simulink model "rev1_PEM"  (R2024a)
settings: Solver=VariableStepAuto  StartTime=0.0  StopTime=10.0  RelTol=1e-3
libraries: spsDiodeLib x2, spsGroundLib x2, spsParallelRLCBranchLib x1, spsControlledVoltageSourceLib x1, spsVariableResistorLib x1
settings Model: Creator=ADMIN  LastModifiedBy=ADMIN

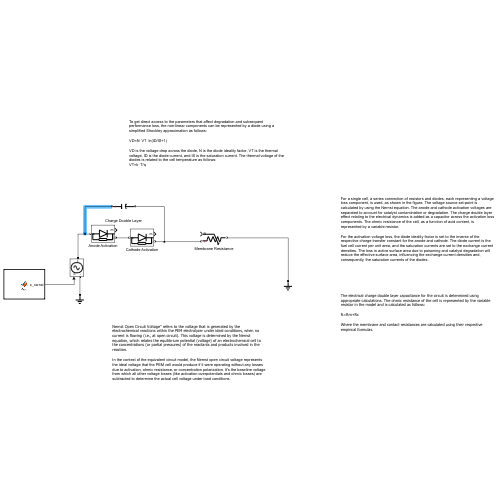
[thumbnail: Simulink's stored preview of the top-level diagram]
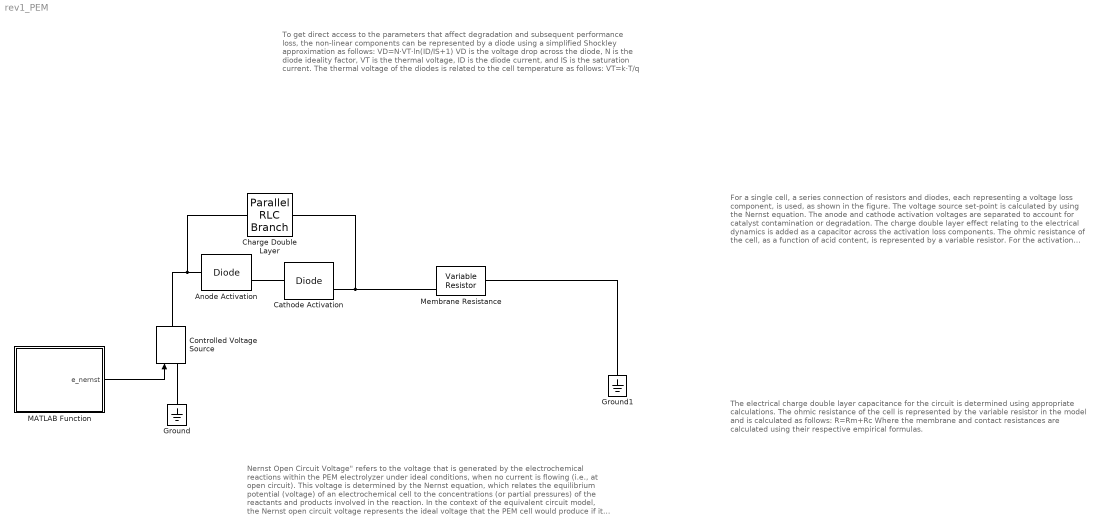
== system rev1_PEM ==
  note: Nernst Open Circuit Voltage" refers to the voltage that is generated by the electrochemical reactions within the PEM electrolyzer under ideal conditions, when no current is flowing (i.e., at open circuit). This voltage is determined by the Nernst equation, which relates the equilibrium potential (voltage) of an electrochemical cell to the concentrations (or partial pressures) of the reactants and products involved in the reaction.
      |
      | In the context of the equivalent circuit model, the Nernst open circuit voltage represents the ideal voltage that the PEM cell would produce if it were operating without any losses due to activation, ohmic resistance, or concentration polarization. It's the baseline voltage from which all other voltage losses (like activation overpotentials and ohmic losses) are subtracted to determine the actual cell voltage under load conditions.
  note: The electrical charge double layer capacitance for the circuit is determined using appropriate calculations. The ohmic resistance of the cell is represented by the variable resistor in the model and is calculated as follows:
      | R=Rm+Rc​
      | Where the membrane and contact resistances are calculated using their respective empirical formulas.
  note: To get direct access to the parameters that affect degradation and subsequent performance loss, the non-linear components can be represented by a diode using a simplified Shockley approximation as follows:
      | VD=N⋅VT⋅ln⁡(ID/IS+1)
      |
      | VD​ is the voltage drop across the diode, N is the diode ideality factor, VT​ is the thermal voltage, ID​ is the diode current, and IS​ is the saturation current. The thermal voltage of the diodes is related to the cell temperature as follows:
      | VT=k⋅T/q
  note: For a single cell, a series connection of resistors and diodes, each representing a voltage loss component, is used, as shown in the figure. The voltage source set-point is calculated by using the Nernst equation. The anode and cathode activation voltages are separated to account for catalyst contamination or degradation. The charge double layer effect relating to the electrical dynamics is added as a capacitor across the activation loss components. The ohmic resistance of the cell, as a function of acid content, is represented by a variable resistor.
      | For the activation voltage loss, the diode ideality factor is set to the inverse of the respective charge transfer constant for the anode and cathode. The diode current is the fuel cell current per unit area, and the saturation currents are set to the exchange current densities. The loss in active surface area due to poisoning and catalyst degradation will reduce the effective surface area, influencing the exchange current densities and, consequently, the saturation currents of the diodes.
  Anode Activation : spsDiodeLib/Diode  Ron=0.001  Lon=0  Vf=0.8  IC=0  UseSnubber=0  Rs=500  Cs=250e-9  Measurements=on
  Cathode Activation : spsDiodeLib/Diode  Ron=0.001  Lon=0  Vf=0.8  IC=0  UseSnubber=0  Rs=500  Cs=250e-9  Measurements=on
  Charge Double Layer : spsParallelRLCBranchLib/Parallel RLC Branch  LConnTagsString=a  RConnTagsString=__new0  BranchType=C  Resistance=1  Inductance=1e-3  SetiL0=off  InitialCurrent=0  Capacitance=1e-6  Setx0=off  InitialVoltage=0  Measurements=None
  Controlled Voltage Source : spsControlledVoltageSourceLib/Controlled Voltage Source  Initialize=on  Source_Type=AC  Amplitude=0  Phase=0  Frequency=0  Measurements=None
  Ground : spsGroundLib/Ground  LConnTagsString=a
  Ground1 : spsGroundLib/Ground  LConnTagsString=a
  MATLAB Function : MATLAB Function  TreatAsAtomicUnit=on
  Membrane Resistance : spsVariableResistorLib/Variable Resistor  Rabsmin=1e-3
      settings: LibrarySourceBlock=sps_lib/Passives/Variable Resistor
  wires:
  MATLAB Function/1(e_nernst) -> Controlled Voltage Source/1
  connections:
  Controlled Voltage Source/LConn1 -- Ground/LConn1
  Membrane Resistance/RConn1 -- Ground1/LConn1
  Anode Activation/RConn1 -- Cathode Activation/LConn1
  Cathode Activation/RConn1 -- Membrane Resistance/LConn1 -- Charge Double Layer/RConn1
  Controlled Voltage Source/RConn1 -- Charge Double Layer/LConn1 -- Anode Activation/LConn1

== matlab function rev1_PEM/MATLAB Function ==
  data: e_nernst output
function e_nernst = fcn()
R = 8.314;         % Universal gas constant in J/(mol*K)
T = 298.15;        % Temperature in Kelvin (e.g., 25°C = 298.15 K)
n = 2;             % Number of electrons transferred in the reaction
F = 96485;         % Faraday's constant in C/mol

% Standard Electrode Potential (example for water splitting)
E_standard = 1.23; % Standard electrode potential in Volts

% Activities (or partial pressures) of reactants and products
a_products = 1; % Activity of products (e.g., partial pressure of oxygen in atm)
a_reactants = 1; % Activity of reactants (e.g., partial pressure of hydrogen in atm)

% Nernst Voltage Calculation
E_nernst = E_standard - (R * T / (n * F)) * log(a_products / a_reactants);
